simulink library "halin"  (R2021b)
settings: Solver=VariableStepAuto  StartTime=0.0  StopTime=10.0  RelTol=1e-3
undefined symbols (not defined in the file): KHAL_CAN1ABM1E2E_flg, KHAL_CAN1EPB1E2E_flg, KHAL_CAN1EPS1E2E_flg, KHAL_CAN1ESC1E2E_flg, KHAL_CAN1ESC5E2E_flg, KHAL_CAN3BMS1E2E_flg, KHAL_CAN3BMS6E2E_flg, KHAL_CAN3CCU1E2E_flg, KHAL_CAN3CCU2E2E_flg, KHAL_CAN3MCUNF1E2E_flg, KHAL_CAN3MCUNR1E2E_flg, KHAL_CAN3Shifter1E2E_flg, KHAL_CAN3Shifter2E2E_flg, KHAL_CAN6FCM2E2E_flg, KHAL_CAN6FCM4E2E_flg, TRUE
libraries: simulink x645, FVT_lib x212, hcu_lib x59
(part 14 of 23)

== system halin/HAL_IN/CAN3/VHAL_CANMsgInvalidMCUNF1_flg ==
  Cast To Boolean13 : DataTypeConversion  OutDataTypeStr=boolean
  Constant : Constant  Value=TRUE
  Latch13 : hcu_lib/Basic_Blocks/Latch
  Switch13 : Switch  Criteria=u2 ~= 0
  Unit Delay : UnitDelay  SampleTime=-1  HasFrameUpgradeWarning=on
  UnitConverter : DataTypeConversion  OutDataTypeStr=boolean
  Out : Outport
  wires:
  Constant/1 -> Switch13/3
  Unit Delay/1 -> Cast To Boolean13/1
  Cast To Boolean13/1 -> Switch13/1, Latch13/1
  Switch13/1 -> UnitConverter/1
  Latch13/1 -> Switch13/2
  UnitConverter/1 -> Unit Delay/1, Out/1  "VHAL_CANMsgInvalidMCUNF1_flg"

== system halin/HAL_IN/CAN3/VHAL_CANMsgInvalidMCUNF2_flg ==
  Cast To Boolean13 : DataTypeConversion  OutDataTypeStr=boolean
  Constant : Constant  Value=TRUE
  Latch13 : hcu_lib/Basic_Blocks/Latch
  Switch13 : Switch  Criteria=u2 ~= 0
  Unit Delay : UnitDelay  SampleTime=-1  HasFrameUpgradeWarning=on
  UnitConverter : DataTypeConversion  OutDataTypeStr=boolean
  Out : Outport
  wires:
  Constant/1 -> Switch13/3
  Unit Delay/1 -> Cast To Boolean13/1
  Cast To Boolean13/1 -> Switch13/1, Latch13/1
  Switch13/1 -> UnitConverter/1
  Latch13/1 -> Switch13/2
  UnitConverter/1 -> Unit Delay/1, Out/1  "VHAL_CANMsgInvalidMCUNF2_flg"

== system halin/HAL_IN/CAN3/VHAL_CANMsgInvalidMCUNF3_flg ==
  Cast To Boolean13 : DataTypeConversion  OutDataTypeStr=boolean
  Constant : Constant  Value=TRUE
  Latch13 : hcu_lib/Basic_Blocks/Latch
  Switch13 : Switch  Criteria=u2 ~= 0
  Unit Delay : UnitDelay  SampleTime=-1  HasFrameUpgradeWarning=on
  UnitConverter : DataTypeConversion  OutDataTypeStr=boolean
  Out : Outport
  wires:
  Constant/1 -> Switch13/3
  Unit Delay/1 -> Cast To Boolean13/1
  Cast To Boolean13/1 -> Switch13/1, Latch13/1
  Switch13/1 -> UnitConverter/1
  Latch13/1 -> Switch13/2
  UnitConverter/1 -> Unit Delay/1, Out/1  "VHAL_CANMsgInvalidMCUNF3_flg"

== system halin/HAL_IN/CAN3/VHAL_CANMsgInvalidMCUNR1_flg ==
  Cast To Boolean13 : DataTypeConversion  OutDataTypeStr=boolean
  Constant : Constant  Value=TRUE
  Latch13 : hcu_lib/Basic_Blocks/Latch
  Switch13 : Switch  Criteria=u2 ~= 0
  Unit Delay : UnitDelay  SampleTime=-1  HasFrameUpgradeWarning=on
  UnitConverter : DataTypeConversion  OutDataTypeStr=boolean
  Out : Outport
  wires:
  Constant/1 -> Switch13/3
  Unit Delay/1 -> Cast To Boolean13/1
  Cast To Boolean13/1 -> Switch13/1, Latch13/1
  Switch13/1 -> UnitConverter/1
  Latch13/1 -> Switch13/2
  UnitConverter/1 -> Unit Delay/1, Out/1  "VHAL_CANMsgInvalidMCUNR1_flg"

== system halin/HAL_IN/CAN3/VHAL_CANMsgInvalidMCUNR2_flg ==
  Cast To Boolean13 : DataTypeConversion  OutDataTypeStr=boolean
  Constant : Constant  Value=TRUE
  Latch13 : hcu_lib/Basic_Blocks/Latch
  Switch13 : Switch  Criteria=u2 ~= 0
  Unit Delay : UnitDelay  SampleTime=-1  HasFrameUpgradeWarning=on
  UnitConverter : DataTypeConversion  OutDataTypeStr=boolean
  Out : Outport
  wires:
  Constant/1 -> Switch13/3
  Unit Delay/1 -> Cast To Boolean13/1
  Cast To Boolean13/1 -> Switch13/1, Latch13/1
  Switch13/1 -> UnitConverter/1
  Latch13/1 -> Switch13/2
  UnitConverter/1 -> Unit Delay/1, Out/1  "VHAL_CANMsgInvalidMCUNR2_flg"

== system halin/HAL_IN/CAN3/VHAL_CANMsgInvalidMCUNR3_flg ==
  Cast To Boolean13 : DataTypeConversion  OutDataTypeStr=boolean
  Constant : Constant  Value=TRUE
  Latch13 : hcu_lib/Basic_Blocks/Latch
  Switch13 : Switch  Criteria=u2 ~= 0
  Unit Delay : UnitDelay  SampleTime=-1  HasFrameUpgradeWarning=on
  UnitConverter : DataTypeConversion  OutDataTypeStr=boolean
  Out : Outport
  wires:
  Constant/1 -> Switch13/3
  Unit Delay/1 -> Cast To Boolean13/1
  Cast To Boolean13/1 -> Switch13/1, Latch13/1
  Switch13/1 -> UnitConverter/1
  Latch13/1 -> Switch13/2
  UnitConverter/1 -> Unit Delay/1, Out/1  "VHAL_CANMsgInvalidMCUNR3_flg"

== system halin/HAL_IN/CAN3/VHAL_CANMsgInvalidShifter1_flg ==
  Cast To Boolean13 : DataTypeConversion  OutDataTypeStr=boolean
  Constant : Constant  Value=TRUE
  Latch13 : hcu_lib/Basic_Blocks/Latch
  Switch13 : Switch  Criteria=u2 ~= 0
  Unit Delay : UnitDelay  SampleTime=-1  HasFrameUpgradeWarning=on
  UnitConverter : DataTypeConversion  OutDataTypeStr=boolean
  Out : Outport
  wires:
  Constant/1 -> Switch13/3
  Unit Delay/1 -> Cast To Boolean13/1
  Cast To Boolean13/1 -> Switch13/1, Latch13/1
  Switch13/1 -> UnitConverter/1
  Latch13/1 -> Switch13/2
  UnitConverter/1 -> Unit Delay/1, Out/1  "VHAL_CANMsgInvalidShifter1_flg"

== system halin/HAL_IN/CAN3/VHAL_CANMsgInvalidShifter2_flg ==
  Cast To Boolean13 : DataTypeConversion  OutDataTypeStr=boolean
  Constant : Constant  Value=TRUE
  Latch13 : hcu_lib/Basic_Blocks/Latch
  Switch13 : Switch  Criteria=u2 ~= 0
  Unit Delay : UnitDelay  SampleTime=-1  HasFrameUpgradeWarning=on
  UnitConverter : DataTypeConversion  OutDataTypeStr=boolean
  Out : Outport
  wires:
  Constant/1 -> Switch13/3
  Unit Delay/1 -> Cast To Boolean13/1
  Cast To Boolean13/1 -> Switch13/1, Latch13/1
  Switch13/1 -> UnitConverter/1
  Latch13/1 -> Switch13/2
  UnitConverter/1 -> Unit Delay/1, Out/1  "VHAL_CANMsgInvalidShifter2_flg"

== system halin/HAL_IN/CAN4/BodyZone_DR1 ==
  DT_CAN4_SG_BodyZone_DR1 : Inport
  BDDSEATAntiSta : Subsystem
  BDDSEATEntryFunSta : Subsystem
  BDDSEATErrorSta : Subsystem
  BDDSEATMemSetSta : Subsystem
  BDDSEATModeSta : Subsystem
  BDDSEATVentSta : Subsystem
  BDDSEATheaterSta : Subsystem
  bus_selector : BusSelector  OutputSignals=CAN4_BD_DSEAT_Anti_Sta
  bus_selector1 : BusSelector  OutputSignals=CAN4_BD_DSEAT_EntryFun_Sta
  bus_selector2 : BusSelector  OutputSignals=CAN4_BD_DSEAT_Error_Sta
  bus_selector3 : BusSelector  OutputSignals=CAN4_BD_DSEAT_MemSet_Sta
  bus_selector4 : BusSelector  OutputSignals=CAN4_BD_DSEAT_Mode_Sta
  bus_selector5 : BusSelector  OutputSignals=CAN4_BD_DSEAT_Vent_Sta
  bus_selector6 : BusSelector  OutputSignals=CAN4_BD_DSEAT_heater_Sta
  VHAL_BDDSEATAntiSta_flg : Outport
  VHAL_BDDSEATEntryFunSta_flg : Outport  Port=2
  VHAL_BDDSEATErrorSta_flg : Outport  Port=3
  VHAL_BDDSEATMemSetSta_enum : Outport  Port=4
  VHAL_BDDSEATModeSta_enum : Outport  Port=5
  VHAL_BDDSEATVentSta_enum : Outport  Port=6
  VHAL_BDDSEATheaterSta_enum : Outport  Port=7
  wires:
  DT_CAN4_SG_BodyZone_DR1/1 -> [DT_CAN4_SG_BodyZone_DR1]
  [DT_CAN4_SG_BodyZone_DR1] -> bus_selector/1
  bus_selector/1 -> BDDSEATAntiSta/1(BD_DSEAT_Anti_Sta)  "<CAN4_BD_DSEAT_Anti_Sta>"
  BDDSEATAntiSta/1(VHAL_BDDSEATAntiSta_flg) -> VHAL_BDDSEATAntiSta_flg/1
  [DT_CAN4_SG_BodyZone_DR1] -> bus_selector1/1
  bus_selector1/1 -> BDDSEATEntryFunSta/1(BD_DSEAT_EntryFun_Sta)  "<CAN4_BD_DSEAT_EntryFun_Sta>"
  BDDSEATEntryFunSta/1(VHAL_BDDSEATEntryFunSta_flg) -> VHAL_BDDSEATEntryFunSta_flg/1
  [DT_CAN4_SG_BodyZone_DR1] -> bus_selector2/1
  bus_selector2/1 -> BDDSEATErrorSta/1(BD_DSEAT_Error_Sta)  "<CAN4_BD_DSEAT_Error_Sta>"
  BDDSEATErrorSta/1(VHAL_BDDSEATErrorSta_flg) -> VHAL_BDDSEATErrorSta_flg/1
  [DT_CAN4_SG_BodyZone_DR1] -> bus_selector3/1
  bus_selector3/1 -> BDDSEATMemSetSta/1(BD_DSEAT_MemSet_Sta)  "<CAN4_BD_DSEAT_MemSet_Sta>"
  BDDSEATMemSetSta/1(VHAL_BDDSEATMemSetSta_enum) -> VHAL_BDDSEATMemSetSta_enum/1
  [DT_CAN4_SG_BodyZone_DR1] -> bus_selector4/1
  bus_selector4/1 -> BDDSEATModeSta/1(BD_DSEAT_Mode_Sta)  "<CAN4_BD_DSEAT_Mode_Sta>"
  BDDSEATModeSta/1(VHAL_BDDSEATModeSta_enum) -> VHAL_BDDSEATModeSta_enum/1
  [DT_CAN4_SG_BodyZone_DR1] -> bus_selector5/1
  bus_selector5/1 -> BDDSEATVentSta/1(BD_DSEAT_Vent_Sta)  "<CAN4_BD_DSEAT_Vent_Sta>"
  BDDSEATVentSta/1(VHAL_BDDSEATVentSta_enum) -> VHAL_BDDSEATVentSta_enum/1
  [DT_CAN4_SG_BodyZone_DR1] -> bus_selector6/1
  bus_selector6/1 -> BDDSEATheaterSta/1(BD_DSEAT_heater_Sta)  "<CAN4_BD_DSEAT_heater_Sta>"
  BDDSEATheaterSta/1(VHAL_BDDSEATheaterSta_enum) -> VHAL_BDDSEATheaterSta_enum/1

== system halin/HAL_IN/CAN4/BodyZone_DR2 ==
  DT_CAN4_SG_BodyZone_DR2 : Inport
  BDAPMWinFOpenedSta : Subsystem
  BDAPMWinROpenedSta : Subsystem
  BDDoorFHandleCloseSta : Subsystem
  BDDoorRHandleCloseSta : Subsystem
  bus_selector : BusSelector  OutputSignals=CAN4_BD_APM_WinFOpened_Sta
  bus_selector1 : BusSelector  OutputSignals=CAN4_BD_APM_WinROpened_Sta
  bus_selector2 : BusSelector  OutputSignals=CAN4_BD_Door_FHandleClose_Sta
  bus_selector3 : BusSelector  OutputSignals=CAN4_BD_Door_RHandleClose_Sta
  VHAL_BDAPMWinFOpenedSta_pct : Outport
  VHAL_BDAPMWinROpenedSta_pct : Outport  Port=2
  VHAL_BDDoorFHandleCloseSta_flg : Outport  Port=3
  VHAL_BDDoorRHandleCloseSta_flg : Outport  Port=4
  wires:
  DT_CAN4_SG_BodyZone_DR2/1 -> [DT_CAN4_SG_BodyZone_DR2]
  [DT_CAN4_SG_BodyZone_DR2] -> bus_selector/1
  bus_selector/1 -> BDAPMWinFOpenedSta/1(BD_APM_WinFOpened_Sta)  "<CAN4_BD_APM_WinFOpened_Sta>"
  BDAPMWinFOpenedSta/1(VHAL_BDAPMWinFOpenedSta_pct) -> VHAL_BDAPMWinFOpenedSta_pct/1
  [DT_CAN4_SG_BodyZone_DR2] -> bus_selector1/1
  bus_selector1/1 -> BDAPMWinROpenedSta/1(BD_APM_WinROpened_Sta)  "<CAN4_BD_APM_WinROpened_Sta>"
  BDAPMWinROpenedSta/1(VHAL_BDAPMWinROpenedSta_pct) -> VHAL_BDAPMWinROpenedSta_pct/1
  [DT_CAN4_SG_BodyZone_DR2] -> bus_selector2/1
  bus_selector2/1 -> BDDoorFHandleCloseSta/1(BD_Door_FHandleClose_Sta)  "<CAN4_BD_Door_FHandleClose_Sta>"
  BDDoorFHandleCloseSta/1(VHAL_BDDoorFHandleCloseSta_flg) -> VHAL_BDDoorFHandleCloseSta_flg/1
  [DT_CAN4_SG_BodyZone_DR2] -> bus_selector3/1
  bus_selector3/1 -> BDDoorRHandleCloseSta/1(BD_Door_RHandleClose_Sta)  "<CAN4_BD_Door_RHandleClose_Sta>"
  BDDoorRHandleCloseSta/1(VHAL_BDDoorRHandleCloseSta_flg) -> VHAL_BDDoorRHandleCloseSta_flg/1

== system halin/HAL_IN/CAN4/BodyZone_PS1 ==
  DT_CAN4_SG_BodyZone_PS1 : Inport
  BPPSEATErrorSta : Subsystem
  BPPSEATModeSta : Subsystem
  BPPSEATVentSta : Subsystem
  BPPSEATheaterSta : Subsystem
  BPPTGActiveSta : Subsystem
  BPPTGExistSta : Subsystem
  BPPTGInsideSW1Sta : Subsystem
  BPPTGInsideSW2Sta : Subsystem
  BPPTGIsSetHeightSta : Subsystem
  BPPTGLeftHallPosnSta : Subsystem
  BPPTGOpenRatioSta : Subsystem
  BPPTGRDILCmd : Subsystem
  BPPTGSysSta : Subsystem
  bus_selector : BusSelector  OutputSignals=CAN4_BP_PSEAT_Error_Sta
  bus_selector1 : BusSelector  OutputSignals=CAN4_BP_PSEAT_Mode_Sta
  bus_selector10 : BusSelector  OutputSignals=CAN4_BP_PTG_OpenRatio_Sta
  bus_selector11 : BusSelector  OutputSignals=CAN4_BP_PTG_RDIL_Cmd
  bus_selector12 : BusSelector  OutputSignals=CAN4_BP_PTG_Sys_Sta
  bus_selector2 : BusSelector  OutputSignals=CAN4_BP_PSEAT_Vent_Sta
  bus_selector3 : BusSelector  OutputSignals=CAN4_BP_PSEAT_heater_Sta
  bus_selector4 : BusSelector  OutputSignals=CAN4_BP_PTG_Active_Sta
  bus_selector5 : BusSelector  OutputSignals=CAN4_BP_PTG_Exist_Sta
  bus_selector6 : BusSelector  OutputSignals=CAN4_BP_PTG_InsideSW1_Sta
  bus_selector7 : BusSelector  OutputSignals=CAN4_BP_PTG_InsideSW2_Sta
  bus_selector8 : BusSelector  OutputSignals=CAN4_BP_PTG_IsSetHeight_Sta
  bus_selector9 : BusSelector  OutputSignals=CAN4_BP_PTG_LeftHallPosn_Sta
  VHAL_BPPSEATErrorSta_flg : Outport
  VHAL_BPPSEATModeSta_enum : Outport  Port=2
  VHAL_BPPSEATVentSta_enum : Outport  Port=3
  VHAL_BPPSEATheaterSta_enum : Outport  Port=4
  VHAL_BPPTGActiveSta_enum : Outport  Port=5
  VHAL_BPPTGExistSta_flg : Outport  Port=6
  VHAL_BPPTGInsideSW1Sta_enum : Outport  Port=7
  VHAL_BPPTGInsideSW2Sta_enum : Outport  Port=8
  VHAL_BPPTGIsSetHeightSta_flg : Outport  Port=9
  VHAL_BPPTGLeftHallPosnSta_enum : Outport  Port=10
  VHAL_BPPTGOpenRatioSta_pct : Outport  Port=11
  VHAL_BPPTGRDILCmd_enum : Outport  Port=12
  VHAL_BPPTGSysSta_enum : Outport  Port=13
  wires:
  DT_CAN4_SG_BodyZone_PS1/1 -> [DT_CAN4_SG_BodyZone_PS1]
  [DT_CAN4_SG_BodyZone_PS1] -> bus_selector/1
  bus_selector/1 -> BPPSEATErrorSta/1(BP_PSEAT_Error_Sta)  "<CAN4_BP_PSEAT_Error_Sta>"
  BPPSEATErrorSta/1(VHAL_BPPSEATErrorSta_flg) -> VHAL_BPPSEATErrorSta_flg/1
  [DT_CAN4_SG_BodyZone_PS1] -> bus_selector1/1
  bus_selector1/1 -> BPPSEATModeSta/1(BP_PSEAT_Mode_Sta)  "<CAN4_BP_PSEAT_Mode_Sta>"
  BPPSEATModeSta/1(VHAL_BPPSEATModeSta_enum) -> VHAL_BPPSEATModeSta_enum/1
  [DT_CAN4_SG_BodyZone_PS1] -> bus_selector2/1
  bus_selector2/1 -> BPPSEATVentSta/1(BP_PSEAT_Vent_Sta)  "<CAN4_BP_PSEAT_Vent_Sta>"
  BPPSEATVentSta/1(VHAL_BPPSEATVentSta_enum) -> VHAL_BPPSEATVentSta_enum/1
  [DT_CAN4_SG_BodyZone_PS1] -> bus_selector3/1
  bus_selector3/1 -> BPPSEATheaterSta/1(BP_PSEAT_heater_Sta)  "<CAN4_BP_PSEAT_heater_Sta>"
  BPPSEATheaterSta/1(VHAL_BPPSEATheaterSta_enum) -> VHAL_BPPSEATheaterSta_enum/1
  [DT_CAN4_SG_BodyZone_PS1] -> bus_selector4/1
  bus_selector4/1 -> BPPTGActiveSta/1(BP_PTG_Active_Sta)  "<CAN4_BP_PTG_Active_Sta>"
  BPPTGActiveSta/1(VHAL_BPPTGActiveSta_enum) -> VHAL_BPPTGActiveSta_enum/1
  [DT_CAN4_SG_BodyZone_PS1] -> bus_selector5/1
  bus_selector5/1 -> BPPTGExistSta/1(BP_PTG_Exist_Sta)  "<CAN4_BP_PTG_Exist_Sta>"
  BPPTGExistSta/1(VHAL_BPPTGExistSta_flg) -> VHAL_BPPTGExistSta_flg/1
  [DT_CAN4_SG_BodyZone_PS1] -> bus_selector6/1
  bus_selector6/1 -> BPPTGInsideSW1Sta/1(BP_PTG_InsideSW1_Sta)  "<CAN4_BP_PTG_InsideSW1_Sta>"
  BPPTGInsideSW1Sta/1(VHAL_BPPTGInsideSW1Sta_enum) -> VHAL_BPPTGInsideSW1Sta_enum/1
  [DT_CAN4_SG_BodyZone_PS1] -> bus_selector7/1
  bus_selector7/1 -> BPPTGInsideSW2Sta/1(BP_PTG_InsideSW2_Sta)  "<CAN4_BP_PTG_InsideSW2_Sta>"
  BPPTGInsideSW2Sta/1(VHAL_BPPTGInsideSW2Sta_enum) -> VHAL_BPPTGInsideSW2Sta_enum/1
  [DT_CAN4_SG_BodyZone_PS1] -> bus_selector8/1
  bus_selector8/1 -> BPPTGIsSetHeightSta/1(BP_PTG_IsSetHeight_Sta)  "<CAN4_BP_PTG_IsSetHeight_Sta>"
  BPPTGIsSetHeightSta/1(VHAL_BPPTGIsSetHeightSta_flg) -> VHAL_BPPTGIsSetHeightSta_flg/1
  [DT_CAN4_SG_BodyZone_PS1] -> bus_selector9/1
  bus_selector9/1 -> BPPTGLeftHallPosnSta/1(BP_PTG_LeftHallPosn_Sta)  "<CAN4_BP_PTG_LeftHallPosn_Sta>"
  BPPTGLeftHallPosnSta/1(VHAL_BPPTGLeftHallPosnSta_enum) -> VHAL_BPPTGLeftHallPosnSta_enum/1
  [DT_CAN4_SG_BodyZone_PS1] -> bus_selector10/1
  bus_selector10/1 -> BPPTGOpenRatioSta/1(BP_PTG_OpenRatio_Sta)  "<CAN4_BP_PTG_OpenRatio_Sta>"
  BPPTGOpenRatioSta/1(VHAL_BPPTGOpenRatioSta_pct) -> VHAL_BPPTGOpenRatioSta_pct/1
  [DT_CAN4_SG_BodyZone_PS1] -> bus_selector11/1
  bus_selector11/1 -> BPPTGRDILCmd/1(BP_PTG_RDIL_Cmd)  "<CAN4_BP_PTG_RDIL_Cmd>"
  BPPTGRDILCmd/1(VHAL_BPPTGRDILCmd_enum) -> VHAL_BPPTGRDILCmd_enum/1
  [DT_CAN4_SG_BodyZone_PS1] -> bus_selector12/1
  bus_selector12/1 -> BPPTGSysSta/1(BP_PTG_Sys_Sta)  "<CAN4_BP_PTG_Sys_Sta>"
  BPPTGSysSta/1(VHAL_BPPTGSysSta_enum) -> VHAL_BPPTGSysSta_enum/1

== system halin/HAL_IN/CAN4/BodyZone_PS2 ==
  DT_CAN4_SG_BodyZone_PS2 : Inport
  BPAPMWinFOpenedSta : Subsystem
  BPAPMWinROpenedSta : Subsystem
  BPDoorFHandleCloseSta : Subsystem
  BPDoorRHandleCloseSta : Subsystem
  BPSEATLVentSta : Subsystem
  BPSEATMLVentSta : Subsystem
  BPSEATMRVentSta : Subsystem
  BPSEATRVentSta : Subsystem
  bus_selector : BusSelector  OutputSignals=CAN4_BP_APM_WinFOpened_Sta
  bus_selector1 : BusSelector  OutputSignals=CAN4_BP_APM_WinROpened_Sta
  bus_selector2 : BusSelector  OutputSignals=CAN4_BP_Door_FHandleClose_Sta
  bus_selector3 : BusSelector  OutputSignals=CAN4_BP_Door_RHandleClose_Sta
  bus_selector4 : BusSelector  OutputSignals=CAN4_BP_SEAT_LVent_Sta
  bus_selector5 : BusSelector  OutputSignals=CAN4_BP_SEAT_MLVent_Sta
  bus_selector6 : BusSelector  OutputSignals=CAN4_BP_SEAT_MRVent_Sta
  bus_selector7 : BusSelector  OutputSignals=CAN4_BP_SEAT_RVent_Sta
  VHAL_BPAPMWinFOpenedSta_pct : Outport
  VHAL_BPAPMWinROpenedSta_pct : Outport  Port=2
  VHAL_BPDoorFHandleCloseSta_flg : Outport  Port=3
  VHAL_BPDoorRHandleCloseSta_flg : Outport  Port=4
  VHAL_BPSEATLVentSta_enum : Outport  Port=5
  VHAL_BPSEATMLVentSta_enum : Outport  Port=6
  VHAL_BPSEATMRVentSta_enum : Outport  Port=7
  VHAL_BPSEATRVentSta_enum : Outport  Port=8
  wires:
  DT_CAN4_SG_BodyZone_PS2/1 -> [DT_CAN4_SG_BodyZone_PS2]
  [DT_CAN4_SG_BodyZone_PS2] -> bus_selector/1
  bus_selector/1 -> BPAPMWinFOpenedSta/1(BP_APM_WinFOpened_Sta)  "<CAN4_BP_APM_WinFOpened_Sta>"
  BPAPMWinFOpenedSta/1(VHAL_BPAPMWinFOpenedSta_pct) -> VHAL_BPAPMWinFOpenedSta_pct/1
  [DT_CAN4_SG_BodyZone_PS2] -> bus_selector1/1
  bus_selector1/1 -> BPAPMWinROpenedSta/1(BP_APM_WinROpened_Sta)  "<CAN4_BP_APM_WinROpened_Sta>"
  BPAPMWinROpenedSta/1(VHAL_BPAPMWinROpenedSta_pct) -> VHAL_BPAPMWinROpenedSta_pct/1
  [DT_CAN4_SG_BodyZone_PS2] -> bus_selector2/1
  bus_selector2/1 -> BPDoorFHandleCloseSta/1(BP_Door_FHandleClose_Sta)  "<CAN4_BP_Door_FHandleClose_Sta>"
  BPDoorFHandleCloseSta/1(VHAL_BPDoorFHandleCloseSta_flg) -> VHAL_BPDoorFHandleCloseSta_flg/1
  [DT_CAN4_SG_BodyZone_PS2] -> bus_selector3/1
  bus_selector3/1 -> BPDoorRHandleCloseSta/1(BP_Door_RHandleClose_Sta)  "<CAN4_BP_Door_RHandleClose_Sta>"
  BPDoorRHandleCloseSta/1(VHAL_BPDoorRHandleCloseSta_flg) -> VHAL_BPDoorRHandleCloseSta_flg/1
  [DT_CAN4_SG_BodyZone_PS2] -> bus_selector4/1
  bus_selector4/1 -> BPSEATLVentSta/1(BP_SEAT_LVent_Sta)  "<CAN4_BP_SEAT_LVent_Sta>"
  BPSEATLVentSta/1(VHAL_BPSEATLVentSta_enum) -> VHAL_BPSEATLVentSta_enum/1
  [DT_CAN4_SG_BodyZone_PS2] -> bus_selector5/1
  bus_selector5/1 -> BPSEATMLVentSta/1(BP_SEAT_MLVent_Sta)  "<CAN4_BP_SEAT_MLVent_Sta>"
  BPSEATMLVentSta/1(VHAL_BPSEATMLVentSta_enum) -> VHAL_BPSEATMLVentSta_enum/1
  [DT_CAN4_SG_BodyZone_PS2] -> bus_selector6/1
  bus_selector6/1 -> BPSEATMRVentSta/1(BP_SEAT_MRVent_Sta)  "<CAN4_BP_SEAT_MRVent_Sta>"
  BPSEATMRVentSta/1(VHAL_BPSEATMRVentSta_enum) -> VHAL_BPSEATMRVentSta_enum/1
  [DT_CAN4_SG_BodyZone_PS2] -> bus_selector7/1
  bus_selector7/1 -> BPSEATRVentSta/1(BP_SEAT_RVent_Sta)  "<CAN4_BP_SEAT_RVent_Sta>"
  BPSEATRVentSta/1(VHAL_BPSEATRVentSta_enum) -> VHAL_BPSEATRVentSta_enum/1

== system halin/HAL_IN/CAN4/DKC1 ==
  DT_CAN4_SG_DKC1 : Inport
  DKCKeyNumSta : Subsystem
  DKCKeyTypeSta : Subsystem
  DKCPDkeyAreaRAPSSta : Subsystem
  DKCParkingModeCmd : Subsystem
  DKCReVehData : Subsystem
  PCommandToBCM : Subsystem
  PCommandToPTG : Subsystem
  PDKeyAreaLockUnlock : Subsystem
  PDKeyAreaPS : Subsystem
  PDKeyAreaPTG : Subsystem
  PDKeyWelcome : Subsystem
  PDkeyShowIVI : Subsystem
  PKeyMiss : Subsystem
  PKeyMode : Subsystem
  PUIDLowPower : Subsystem
  bus_selector : BusSelector  OutputSignals=CAN4_DKC_KeyNum_Sta
  bus_selector1 : BusSelector  OutputSignals=CAN4_DKC_KeyType_Sta
  bus_selector10 : BusSelector  OutputSignals=CAN4_P_DKey_Welcome
  bus_selector11 : BusSelector  OutputSignals=CAN4_P_Dkey_Show_IVI
  bus_selector12 : BusSelector  OutputSignals=CAN4_P_KeyMiss
  bus_selector13 : BusSelector  OutputSignals=CAN4_P_KeyMode
  bus_selector14 : BusSelector  OutputSignals=CAN4_P_UID_LowPower
  bus_selector2 : BusSelector  OutputSignals=CAN4_DKC_PDkeyAreaRAPS_Sta
  bus_selector3 : BusSelector  OutputSignals=CAN4_DKC_ParkingMode_Cmd
  bus_selector4 : BusSelector  OutputSignals=CAN4_DKC_Re_VehData
  bus_selector5 : BusSelector  OutputSignals=CAN4_P_CommandToBCM
  bus_selector6 : BusSelector  OutputSignals=CAN4_P_CommandToPTG
  bus_selector7 : BusSelector  OutputSignals=CAN4_P_DKey_Area_LockUnlock
  bus_selector8 : BusSelector  OutputSignals=CAN4_P_DKey_Area_PS
  bus_selector9 : BusSelector  OutputSignals=CAN4_P_DKey_Area_PTG
  VHAL_DKCKeyNumSta_enum : Outport
  VHAL_DKCKeyTypeSta_enum : Outport  Port=2
  VHAL_DKCPDkeyAreaRAPSSta_enum : Outport  Port=3
  VHAL_DKCParkingModeCmd_enum : Outport  Port=4
  VHAL_DKCReVehData_enum : Outport  Port=5
  VHAL_PCommandToBCM_enum : Outport  Port=6
  VHAL_PCommandToPTG_enum : Outport  Port=7
  VHAL_PDKeyAreaLockUnlock_enum : Outport  Port=8
  VHAL_PDKeyAreaPS_enum : Outport  Port=9
  VHAL_PDKeyAreaPTG_enum : Outport  Port=10
  VHAL_PDKeyWelcome_enum : Outport  Port=11
  VHAL_PDkeyShowIVI_enum : Outport  Port=12
  VHAL_PKeyMiss_flg : Outport  Port=13
  VHAL_PKeyMode_enum : Outport  Port=14
  VHAL_PUIDLowPower_flg : Outport  Port=15
  wires:
  DT_CAN4_SG_DKC1/1 -> [DT_CAN4_SG_DKC1]
  [DT_CAN4_SG_DKC1] -> bus_selector/1
  bus_selector/1 -> DKCKeyNumSta/1(DKC_KeyNum_Sta)  "<CAN4_DKC_KeyNum_Sta>"
  DKCKeyNumSta/1(VHAL_DKCKeyNumSta_enum) -> VHAL_DKCKeyNumSta_enum/1
  [DT_CAN4_SG_DKC1] -> bus_selector1/1
  bus_selector1/1 -> DKCKeyTypeSta/1(DKC_KeyType_Sta)  "<CAN4_DKC_KeyType_Sta>"
  DKCKeyTypeSta/1(VHAL_DKCKeyTypeSta_enum) -> VHAL_DKCKeyTypeSta_enum/1
  [DT_CAN4_SG_DKC1] -> bus_selector2/1
  bus_selector2/1 -> DKCPDkeyAreaRAPSSta/1(DKC_PDkeyAreaRAPS_Sta)  "<CAN4_DKC_PDkeyAreaRAPS_Sta>"
  DKCPDkeyAreaRAPSSta/1(VHAL_DKCPDkeyAreaRAPSSta_enum) -> VHAL_DKCPDkeyAreaRAPSSta_enum/1
  [DT_CAN4_SG_DKC1] -> bus_selector3/1
  bus_selector3/1 -> DKCParkingModeCmd/1(DKC_ParkingMode_Cmd)  "<CAN4_DKC_ParkingMode_Cmd>"
  DKCParkingModeCmd/1(VHAL_DKCParkingModeCmd_enum) -> VHAL_DKCParkingModeCmd_enum/1
  [DT_CAN4_SG_DKC1] -> bus_selector4/1
  bus_selector4/1 -> DKCReVehData/1(DKC_Re_VehData)  "<CAN4_DKC_Re_VehData>"
  DKCReVehData/1(VHAL_DKCReVehData_enum) -> VHAL_DKCReVehData_enum/1
  [DT_CAN4_SG_DKC1] -> bus_selector5/1
  bus_selector5/1 -> PCommandToBCM/1(P_CommandToBCM)  "<CAN4_P_CommandToBCM>"
  PCommandToBCM/1(VHAL_PCommandToBCM_enum) -> VHAL_PCommandToBCM_enum/1
  [DT_CAN4_SG_DKC1] -> bus_selector6/1
  bus_selector6/1 -> PCommandToPTG/1(P_CommandToPTG)  "<CAN4_P_CommandToPTG>"
  PCommandToPTG/1(VHAL_PCommandToPTG_enum) -> VHAL_PCommandToPTG_enum/1
  [DT_CAN4_SG_DKC1] -> bus_selector7/1
  bus_selector7/1 -> PDKeyAreaLockUnlock/1(P_DKey_Area_LockUnlock)  "<CAN4_P_DKey_Area_LockUnlock>"
  PDKeyAreaLockUnlock/1(VHAL_PDKeyAreaLockUnlock_enum) -> VHAL_PDKeyAreaLockUnlock_enum/1
  [DT_CAN4_SG_DKC1] -> bus_selector8/1
  bus_selector8/1 -> PDKeyAreaPS/1(P_DKey_Area_PS)  "<CAN4_P_DKey_Area_PS>"
  PDKeyAreaPS/1(VHAL_PDKeyAreaPS_enum) -> VHAL_PDKeyAreaPS_enum/1
  [DT_CAN4_SG_DKC1] -> bus_selector9/1
  bus_selector9/1 -> PDKeyAreaPTG/1(P_DKey_Area_PTG)  "<CAN4_P_DKey_Area_PTG>"
  PDKeyAreaPTG/1(VHAL_PDKeyAreaPTG_enum) -> VHAL_PDKeyAreaPTG_enum/1
  [DT_CAN4_SG_DKC1] -> bus_selector10/1
  bus_selector10/1 -> PDKeyWelcome/1(P_DKey_Welcome)  "<CAN4_P_DKey_Welcome>"
  PDKeyWelcome/1(VHAL_PDKeyWelcome_enum) -> VHAL_PDKeyWelcome_enum/1
  [DT_CAN4_SG_DKC1] -> bus_selector11/1
  bus_selector11/1 -> PDkeyShowIVI/1(P_Dkey_Show_IVI)  "<CAN4_P_Dkey_Show_IVI>"
  PDkeyShowIVI/1(VHAL_PDkeyShowIVI_enum) -> VHAL_PDkeyShowIVI_enum/1
  [DT_CAN4_SG_DKC1] -> bus_selector12/1
  bus_selector12/1 -> PKeyMiss/1(P_KeyMiss)  "<CAN4_P_KeyMiss>"
  PKeyMiss/1(VHAL_PKeyMiss_flg) -> VHAL_PKeyMiss_flg/1
  [DT_CAN4_SG_DKC1] -> bus_selector13/1
  bus_selector13/1 -> PKeyMode/1(P_KeyMode)  "<CAN4_P_KeyMode>"
  PKeyMode/1(VHAL_PKeyMode_enum) -> VHAL_PKeyMode_enum/1
  [DT_CAN4_SG_DKC1] -> bus_selector14/1
  bus_selector14/1 -> PUIDLowPower/1(P_UID_LowPower)  "<CAN4_P_UID_LowPower>"
  PUIDLowPower/1(VHAL_PUIDLowPower_flg) -> VHAL_PUIDLowPower_flg/1

== system halin/HAL_IN/CAN4/DKC2 ==
  DT_CAN4_SG_DKC2 : Inport
  EncryptionDATA063 : Subsystem
  EncryptionDATA64127 : Subsystem
  RandomNumberX : Subsystem
  bus_selector : BusSelector  OutputSignals=CAN4_EncryptionDATA_0_63
  bus_selector1 : BusSelector  OutputSignals=CAN4_EncryptionDATA_64_127
  bus_selector2 : BusSelector  OutputSignals=CAN4_Random_Number_X
  VHAL_EncryptionDATA063_enum : Outport
  VHAL_EncryptionDATA64127_enum : Outport  Port=2
  VHAL_RandomNumberX_enum : Outport  Port=3
  wires:
  DT_CAN4_SG_DKC2/1 -> [DT_CAN4_SG_DKC2]
  [DT_CAN4_SG_DKC2] -> bus_selector/1
  bus_selector/1 -> EncryptionDATA063/1(EncryptionDATA_0_63)  "<CAN4_EncryptionDATA_0_63>"
  EncryptionDATA063/1(VHAL_EncryptionDATA063_enum) -> VHAL_EncryptionDATA063_enum/1
  [DT_CAN4_SG_DKC2] -> bus_selector1/1
  bus_selector1/1 -> EncryptionDATA64127/1(EncryptionDATA_64_127)  "<CAN4_EncryptionDATA_64_127>"
  EncryptionDATA64127/1(VHAL_EncryptionDATA64127_enum) -> VHAL_EncryptionDATA64127_enum/1
  [DT_CAN4_SG_DKC2] -> bus_selector2/1
  bus_selector2/1 -> RandomNumberX/1(Random_Number_X)  "<CAN4_Random_Number_X>"
  RandomNumberX/1(VHAL_RandomNumberX_enum) -> VHAL_RandomNumberX_enum/1

== system halin/HAL_IN/CAN4/PTG1 ==
  DT_CAN4_SG_PTG1 : Inport
  PTGActiveSta : Subsystem
  PTGAutoStaus : Subsystem
  PTGExist : Subsystem
  PTGHWVer : Subsystem
  PTGInnerSW2 : Subsystem
  PTGIsSetHeight : Subsystem
  PTGOpenRatio : Subsystem
  PTGRDILSta : Subsystem
  PTGSWVer : Subsystem
  PTGSysSta : Subsystem
  bus_selector : BusSelector  OutputSignals=CAN4_PTG_Active_Sta
  bus_selector1 : BusSelector  OutputSignals=CAN4_PTG_AutoStaus
  bus_selector2 : BusSelector  OutputSignals=CAN4_PTG_Exist
  bus_selector3 : BusSelector  OutputSignals=CAN4_PTG_HW_Ver
  bus_selector4 : BusSelector  OutputSignals=CAN4_PTG_Inner_SW_2
  bus_selector5 : BusSelector  OutputSignals=CAN4_PTG_Is_Set_Height
  bus_selector6 : BusSelector  OutputSignals=CAN4_PTG_Open_Ratio
  bus_selector7 : BusSelector  OutputSignals=CAN4_PTG_RDIL_Sta
  bus_selector8 : BusSelector  OutputSignals=CAN4_PTG_SW_Ver
  bus_selector9 : BusSelector  OutputSignals=CAN4_PTG_Sys_Sta
  VHAL_PTGActiveSta_enum : Outport
  VHAL_PTGAutoStaus_flg : Outport  Port=2
  VHAL_PTGExist_flg : Outport  Port=3
  VHAL_PTGHWVer_enum : Outport  Port=4
  VHAL_PTGInnerSW2_enum : Outport  Port=5
  VHAL_PTGIsSetHeight_flg : Outport  Port=6
  VHAL_PTGOpenRatio_pct : Outport  Port=7
  VHAL_PTGRDILSta_enum : Outport  Port=8
  VHAL_PTGSWVer_enum : Outport  Port=9
  VHAL_PTGSysSta_enum : Outport  Port=10
  wires:
  DT_CAN4_SG_PTG1/1 -> [DT_CAN4_SG_PTG1]
  [DT_CAN4_SG_PTG1] -> bus_selector/1
  bus_selector/1 -> PTGActiveSta/1(PTG_Active_Sta)  "<CAN4_PTG_Active_Sta>"
  PTGActiveSta/1(VHAL_PTGActiveSta_enum) -> VHAL_PTGActiveSta_enum/1
  [DT_CAN4_SG_PTG1] -> bus_selector1/1
  bus_selector1/1 -> PTGAutoStaus/1(PTG_AutoStaus)  "<CAN4_PTG_AutoStaus>"
  PTGAutoStaus/1(VHAL_PTGAutoStaus_flg) -> VHAL_PTGAutoStaus_flg/1
  [DT_CAN4_SG_PTG1] -> bus_selector2/1
  bus_selector2/1 -> PTGExist/1(PTG_Exist)  "<CAN4_PTG_Exist>"
  PTGExist/1(VHAL_PTGExist_flg) -> VHAL_PTGExist_flg/1
  [DT_CAN4_SG_PTG1] -> bus_selector3/1
  bus_selector3/1 -> PTGHWVer/1(PTG_HW_Ver)  "<CAN4_PTG_HW_Ver>"
  PTGHWVer/1(VHAL_PTGHWVer_enum) -> VHAL_PTGHWVer_enum/1
  [DT_CAN4_SG_PTG1] -> bus_selector4/1
  bus_selector4/1 -> PTGInnerSW2/1(PTG_Inner_SW_2)  "<CAN4_PTG_Inner_SW_2>"
  PTGInnerSW2/1(VHAL_PTGInnerSW2_enum) -> VHAL_PTGInnerSW2_enum/1
  [DT_CAN4_SG_PTG1] -> bus_selector5/1
  bus_selector5/1 -> PTGIsSetHeight/1(PTG_Is_Set_Height)  "<CAN4_PTG_Is_Set_Height>"
  PTGIsSetHeight/1(VHAL_PTGIsSetHeight_flg) -> VHAL_PTGIsSetHeight_flg/1
  [DT_CAN4_SG_PTG1] -> bus_selector6/1
  bus_selector6/1 -> PTGOpenRatio/1(PTG_Open_Ratio)  "<CAN4_PTG_Open_Ratio>"
  PTGOpenRatio/1(VHAL_PTGOpenRatio_pct) -> VHAL_PTGOpenRatio_pct/1
  [DT_CAN4_SG_PTG1] -> bus_selector7/1
  bus_selector7/1 -> PTGRDILSta/1(PTG_RDIL_Sta)  "<CAN4_PTG_RDIL_Sta>"
  PTGRDILSta/1(VHAL_PTGRDILSta_enum) -> VHAL_PTGRDILSta_enum/1
  [DT_CAN4_SG_PTG1] -> bus_selector8/1
  bus_selector8/1 -> PTGSWVer/1(PTG_SW_Ver)  "<CAN4_PTG_SW_Ver>"
  PTGSWVer/1(VHAL_PTGSWVer_enum) -> VHAL_PTGSWVer_enum/1
  [DT_CAN4_SG_PTG1] -> bus_selector9/1
  bus_selector9/1 -> PTGSysSta/1(PTG_Sys_Sta)  "<CAN4_PTG_Sys_Sta>"
  PTGSysSta/1(VHAL_PTGSysSta_enum) -> VHAL_PTGSysSta_enum/1

== system halin/HAL_IN/CAN4/VHAL_CANMsgInvalidBodyZoneDR1_flg ==
  Cast To Boolean13 : DataTypeConversion  OutDataTypeStr=boolean
  Constant : Constant  Value=TRUE
  Latch13 : hcu_lib/Basic_Blocks/Latch
  Switch13 : Switch  Criteria=u2 ~= 0
  Unit Delay : UnitDelay  SampleTime=-1  HasFrameUpgradeWarning=on
  UnitConverter : DataTypeConversion  OutDataTypeStr=boolean
  Out : Outport
  wires:
  Constant/1 -> Switch13/3
  Unit Delay/1 -> Cast To Boolean13/1
  Cast To Boolean13/1 -> Switch13/1, Latch13/1
  Switch13/1 -> UnitConverter/1
  Latch13/1 -> Switch13/2
  UnitConverter/1 -> Unit Delay/1, Out/1  "VHAL_CANMsgInvalidBodyZoneDR1_flg"

== system halin/HAL_IN/CAN4/VHAL_CANMsgInvalidBodyZoneDR2_flg ==
  Cast To Boolean13 : DataTypeConversion  OutDataTypeStr=boolean
  Constant : Constant  Value=TRUE
  Latch13 : hcu_lib/Basic_Blocks/Latch
  Switch13 : Switch  Criteria=u2 ~= 0
  Unit Delay : UnitDelay  SampleTime=-1  HasFrameUpgradeWarning=on
  UnitConverter : DataTypeConversion  OutDataTypeStr=boolean
  Out : Outport
  wires:
  Constant/1 -> Switch13/3
  Unit Delay/1 -> Cast To Boolean13/1
  Cast To Boolean13/1 -> Switch13/1, Latch13/1
  Switch13/1 -> UnitConverter/1
  Latch13/1 -> Switch13/2
  UnitConverter/1 -> Unit Delay/1, Out/1  "VHAL_CANMsgInvalidBodyZoneDR2_flg"

== system halin/HAL_IN/CAN4/VHAL_CANMsgInvalidBodyZonePS1_flg ==
  Cast To Boolean13 : DataTypeConversion  OutDataTypeStr=boolean
  Constant : Constant  Value=TRUE
  Latch13 : hcu_lib/Basic_Blocks/Latch
  Switch13 : Switch  Criteria=u2 ~= 0
  Unit Delay : UnitDelay  SampleTime=-1  HasFrameUpgradeWarning=on
  UnitConverter : DataTypeConversion  OutDataTypeStr=boolean
  Out : Outport
  wires:
  Constant/1 -> Switch13/3
  Unit Delay/1 -> Cast To Boolean13/1
  Cast To Boolean13/1 -> Switch13/1, Latch13/1
  Switch13/1 -> UnitConverter/1
  Latch13/1 -> Switch13/2
  UnitConverter/1 -> Unit Delay/1, Out/1  "VHAL_CANMsgInvalidBodyZonePS1_flg"

== system halin/HAL_IN/CAN4/VHAL_CANMsgInvalidBodyZonePS2_flg ==
  Cast To Boolean13 : DataTypeConversion  OutDataTypeStr=boolean
  Constant : Constant  Value=TRUE
  Latch13 : hcu_lib/Basic_Blocks/Latch
  Switch13 : Switch  Criteria=u2 ~= 0
  Unit Delay : UnitDelay  SampleTime=-1  HasFrameUpgradeWarning=on
  UnitConverter : DataTypeConversion  OutDataTypeStr=boolean
  Out : Outport
  wires:
  Constant/1 -> Switch13/3
  Unit Delay/1 -> Cast To Boolean13/1
  Cast To Boolean13/1 -> Switch13/1, Latch13/1
  Switch13/1 -> UnitConverter/1
  Latch13/1 -> Switch13/2
  UnitConverter/1 -> Unit Delay/1, Out/1  "VHAL_CANMsgInvalidBodyZonePS2_flg"

== system halin/HAL_IN/CAN4/VHAL_CANMsgInvalidDKC1_flg ==
  Cast To Boolean13 : DataTypeConversion  OutDataTypeStr=boolean
  Constant : Constant  Value=TRUE
  Latch13 : hcu_lib/Basic_Blocks/Latch
  Switch13 : Switch  Criteria=u2 ~= 0
  Unit Delay : UnitDelay  SampleTime=-1  HasFrameUpgradeWarning=on
  UnitConverter : DataTypeConversion  OutDataTypeStr=boolean
  Out : Outport
  wires:
  Constant/1 -> Switch13/3
  Unit Delay/1 -> Cast To Boolean13/1
  Cast To Boolean13/1 -> Switch13/1, Latch13/1
  Switch13/1 -> UnitConverter/1
  Latch13/1 -> Switch13/2
  UnitConverter/1 -> Unit Delay/1, Out/1  "VHAL_CANMsgInvalidDKC1_flg"

== system halin/HAL_IN/CAN4/VHAL_CANMsgInvalidDKC2_flg ==
  Cast To Boolean13 : DataTypeConversion  OutDataTypeStr=boolean
  Constant : Constant  Value=TRUE
  Latch13 : hcu_lib/Basic_Blocks/Latch
  Switch13 : Switch  Criteria=u2 ~= 0
  Unit Delay : UnitDelay  SampleTime=-1  HasFrameUpgradeWarning=on
  UnitConverter : DataTypeConversion  OutDataTypeStr=boolean
  Out : Outport
  wires:
  Constant/1 -> Switch13/3
  Unit Delay/1 -> Cast To Boolean13/1
  Cast To Boolean13/1 -> Switch13/1, Latch13/1
  Switch13/1 -> UnitConverter/1
  Latch13/1 -> Switch13/2
  UnitConverter/1 -> Unit Delay/1, Out/1  "VHAL_CANMsgInvalidDKC2_flg"

== system halin/HAL_IN/CAN4/VHAL_CANMsgInvalidPTG1_flg ==
  Cast To Boolean13 : DataTypeConversion  OutDataTypeStr=boolean
  Constant : Constant  Value=TRUE
  Latch13 : hcu_lib/Basic_Blocks/Latch
  Switch13 : Switch  Criteria=u2 ~= 0
  Unit Delay : UnitDelay  SampleTime=-1  HasFrameUpgradeWarning=on
  UnitConverter : DataTypeConversion  OutDataTypeStr=boolean
  Out : Outport
  wires:
  Constant/1 -> Switch13/3
  Unit Delay/1 -> Cast To Boolean13/1
  Cast To Boolean13/1 -> Switch13/1, Latch13/1
  Switch13/1 -> UnitConverter/1
  Latch13/1 -> Switch13/2
  UnitConverter/1 -> Unit Delay/1, Out/1  "VHAL_CANMsgInvalidPTG1_flg"

== system halin/HAL_IN/CAN4/VHAL_CANMsgInvalidZONEDR1_flg ==
  Cast To Boolean13 : DataTypeConversion  OutDataTypeStr=boolean
  Constant : Constant  Value=TRUE
  Latch13 : hcu_lib/Basic_Blocks/Latch
  Switch13 : Switch  Criteria=u2 ~= 0
  Unit Delay : UnitDelay  SampleTime=-1  HasFrameUpgradeWarning=on
  UnitConverter : DataTypeConversion  OutDataTypeStr=boolean
  Out : Outport
  wires:
  Constant/1 -> Switch13/3
  Unit Delay/1 -> Cast To Boolean13/1
  Cast To Boolean13/1 -> Switch13/1, Latch13/1
  Switch13/1 -> UnitConverter/1
  Latch13/1 -> Switch13/2
  UnitConverter/1 -> Unit Delay/1, Out/1  "VHAL_CANMsgInvalidZONEDR1_flg"

== system halin/HAL_IN/CAN4/VHAL_CANMsgInvalidZONEDRVCU_flg ==
  Cast To Boolean13 : DataTypeConversion  OutDataTypeStr=boolean
  Constant : Constant  Value=TRUE
  Latch13 : hcu_lib/Basic_Blocks/Latch
  Switch13 : Switch  Criteria=u2 ~= 0
  Unit Delay : UnitDelay  SampleTime=-1  HasFrameUpgradeWarning=on
  UnitConverter : DataTypeConversion  OutDataTypeStr=boolean
  Out : Outport
  wires:
  Constant/1 -> Switch13/3
  Unit Delay/1 -> Cast To Boolean13/1
  Cast To Boolean13/1 -> Switch13/1, Latch13/1
  Switch13/1 -> UnitConverter/1
  Latch13/1 -> Switch13/2
  UnitConverter/1 -> Unit Delay/1, Out/1  "VHAL_CANMsgInvalidZONEDRVCU_flg"

== system halin/HAL_IN/CAN4/VHAL_CANMsgInvalidZONEFR1_flg ==
  Cast To Boolean13 : DataTypeConversion  OutDataTypeStr=boolean
  Constant : Constant  Value=TRUE
  Latch13 : hcu_lib/Basic_Blocks/Latch
  Switch13 : Switch  Criteria=u2 ~= 0
  Unit Delay : UnitDelay  SampleTime=-1  HasFrameUpgradeWarning=on
  UnitConverter : DataTypeConversion  OutDataTypeStr=boolean
  Out : Outport
  wires:
  Constant/1 -> Switch13/3
  Unit Delay/1 -> Cast To Boolean13/1
  Cast To Boolean13/1 -> Switch13/1, Latch13/1
  Switch13/1 -> UnitConverter/1
  Latch13/1 -> Switch13/2
  UnitConverter/1 -> Unit Delay/1, Out/1  "VHAL_CANMsgInvalidZONEFR1_flg"

== system halin/HAL_IN/CAN4/VHAL_CANMsgInvalidZONEFRVCU_flg ==
  Cast To Boolean13 : DataTypeConversion  OutDataTypeStr=boolean
  Constant : Constant  Value=TRUE
  Latch13 : hcu_lib/Basic_Blocks/Latch
  Switch13 : Switch  Criteria=u2 ~= 0
  Unit Delay : UnitDelay  SampleTime=-1  HasFrameUpgradeWarning=on
  UnitConverter : DataTypeConversion  OutDataTypeStr=boolean
  Out : Outport
  wires:
  Constant/1 -> Switch13/3
  Unit Delay/1 -> Cast To Boolean13/1
  Cast To Boolean13/1 -> Switch13/1, Latch13/1
  Switch13/1 -> UnitConverter/1
  Latch13/1 -> Switch13/2
  UnitConverter/1 -> Unit Delay/1, Out/1  "VHAL_CANMsgInvalidZONEFRVCU_flg"

== system halin/HAL_IN/CAN4/VHAL_CANMsgInvalidzGWAPTC1_flg ==
  Cast To Boolean13 : DataTypeConversion  OutDataTypeStr=boolean
  Constant : Constant  Value=TRUE
  Latch13 : hcu_lib/Basic_Blocks/Latch
  Switch13 : Switch  Criteria=u2 ~= 0
  Unit Delay : UnitDelay  SampleTime=-1  HasFrameUpgradeWarning=on
  UnitConverter : DataTypeConversion  OutDataTypeStr=boolean
  Out : Outport
  wires:
  Constant/1 -> Switch13/3
  Unit Delay/1 -> Cast To Boolean13/1
  Cast To Boolean13/1 -> Switch13/1, Latch13/1
  Switch13/1 -> UnitConverter/1
  Latch13/1 -> Switch13/2
  UnitConverter/1 -> Unit Delay/1, Out/1  "VHAL_CANMsgInvalidzGWAPTC1_flg"

== system halin/HAL_IN/CAN4/VHAL_CANMsgInvalidzGWCANFr1_flg ==
  Cast To Boolean13 : DataTypeConversion  OutDataTypeStr=boolean
  Constant : Constant  Value=TRUE
  Latch13 : hcu_lib/Basic_Blocks/Latch
  Switch13 : Switch  Criteria=u2 ~= 0
  Unit Delay : UnitDelay  SampleTime=-1  HasFrameUpgradeWarning=on
  UnitConverter : DataTypeConversion  OutDataTypeStr=boolean
  Out : Outport
  wires:
  Constant/1 -> Switch13/3
  Unit Delay/1 -> Cast To Boolean13/1
  Cast To Boolean13/1 -> Switch13/1, Latch13/1
  Switch13/1 -> UnitConverter/1
  Latch13/1 -> Switch13/2
  UnitConverter/1 -> Unit Delay/1, Out/1  "VHAL_CANMsgInvalidzGWCANFr1_flg"

== system halin/HAL_IN/CAN4/VHAL_CANMsgInvalidzGWLINDr1_flg ==
  Cast To Boolean13 : DataTypeConversion  OutDataTypeStr=boolean
  Constant : Constant  Value=TRUE
  Latch13 : hcu_lib/Basic_Blocks/Latch
  Switch13 : Switch  Criteria=u2 ~= 0
  Unit Delay : UnitDelay  SampleTime=-1  HasFrameUpgradeWarning=on
  UnitConverter : DataTypeConversion  OutDataTypeStr=boolean
  Out : Outport
  wires:
  Constant/1 -> Switch13/3
  Unit Delay/1 -> Cast To Boolean13/1
  Cast To Boolean13/1 -> Switch13/1, Latch13/1
  Switch13/1 -> UnitConverter/1
  Latch13/1 -> Switch13/2
  UnitConverter/1 -> Unit Delay/1, Out/1  "VHAL_CANMsgInvalidzGWLINDr1_flg"

== system halin/HAL_IN/CAN4/VHAL_CANMsgInvalidzGWLINDr2_flg ==
  Cast To Boolean13 : DataTypeConversion  OutDataTypeStr=boolean
  Constant : Constant  Value=TRUE
  Latch13 : hcu_lib/Basic_Blocks/Latch
  Switch13 : Switch  Criteria=u2 ~= 0
  Unit Delay : UnitDelay  SampleTime=-1  HasFrameUpgradeWarning=on
  UnitConverter : DataTypeConversion  OutDataTypeStr=boolean
  Out : Outport
  wires:
  Constant/1 -> Switch13/3
  Unit Delay/1 -> Cast To Boolean13/1
  Cast To Boolean13/1 -> Switch13/1, Latch13/1
  Switch13/1 -> UnitConverter/1
  Latch13/1 -> Switch13/2
  UnitConverter/1 -> Unit Delay/1, Out/1  "VHAL_CANMsgInvalidzGWLINDr2_flg"

== system halin/HAL_IN/CAN4/VHAL_CANMsgInvalidzGWLINFr1_flg ==
  Cast To Boolean13 : DataTypeConversion  OutDataTypeStr=boolean
  Constant : Constant  Value=TRUE
  Latch13 : hcu_lib/Basic_Blocks/Latch
  Switch13 : Switch  Criteria=u2 ~= 0
  Unit Delay : UnitDelay  SampleTime=-1  HasFrameUpgradeWarning=on
  UnitConverter : DataTypeConversion  OutDataTypeStr=boolean
  Out : Outport
  wires:
  Constant/1 -> Switch13/3
  Unit Delay/1 -> Cast To Boolean13/1
  Cast To Boolean13/1 -> Switch13/1, Latch13/1
  Switch13/1 -> UnitConverter/1
  Latch13/1 -> Switch13/2
  UnitConverter/1 -> Unit Delay/1, Out/1  "VHAL_CANMsgInvalidzGWLINFr1_flg"

== system halin/HAL_IN/CAN4/VHAL_CANMsgInvalidzGWLINFr2_flg ==
  Cast To Boolean13 : DataTypeConversion  OutDataTypeStr=boolean
  Constant : Constant  Value=TRUE
  Latch13 : hcu_lib/Basic_Blocks/Latch
  Switch13 : Switch  Criteria=u2 ~= 0
  Unit Delay : UnitDelay  SampleTime=-1  HasFrameUpgradeWarning=on
  UnitConverter : DataTypeConversion  OutDataTypeStr=boolean
  Out : Outport
  wires:
  Constant/1 -> Switch13/3
  Unit Delay/1 -> Cast To Boolean13/1
  Cast To Boolean13/1 -> Switch13/1, Latch13/1
  Switch13/1 -> UnitConverter/1
  Latch13/1 -> Switch13/2
  UnitConverter/1 -> Unit Delay/1, Out/1  "VHAL_CANMsgInvalidzGWLINFr2_flg"

== system halin/HAL_IN/CAN4/VHAL_CANMsgInvalidzGWSEAT1_flg ==
  Cast To Boolean13 : DataTypeConversion  OutDataTypeStr=boolean
  Constant : Constant  Value=TRUE
  Latch13 : hcu_lib/Basic_Blocks/Latch
  Switch13 : Switch  Criteria=u2 ~= 0
  Unit Delay : UnitDelay  SampleTime=-1  HasFrameUpgradeWarning=on
  UnitConverter : DataTypeConversion  OutDataTypeStr=boolean
  Out : Outport
  wires:
  Constant/1 -> Switch13/3
  Unit Delay/1 -> Cast To Boolean13/1
  Cast To Boolean13/1 -> Switch13/1, Latch13/1
  Switch13/1 -> UnitConverter/1
  Latch13/1 -> Switch13/2
  UnitConverter/1 -> Unit Delay/1, Out/1  "VHAL_CANMsgInvalidzGWSEAT1_flg"

== system halin/HAL_IN/CAN4/ZONE_DR1 ==
  DT_CAN4_SG_ZONE_DR1 : Inport
  DrLockSta : Subsystem
  MIRRORFOLDSW : Subsystem
  RLTurnLPErr : Subsystem
  RLTurnLampC : Subsystem
  RRTurnLPErr : Subsystem
  RRTurnLampC : Subsystem
  RWiperAS : Subsystem
  RWiperProtection : Subsystem
  bus_selector : BusSelector  OutputSignals=CAN4_DrLockSta
  bus_selector1 : BusSelector  OutputSignals=CAN4_MIRROR_FOLD_SW
  bus_selector2 : BusSelector  OutputSignals=CAN4_RLTurnLPErr
  bus_selector3 : BusSelector  OutputSignals=CAN4_RLTurnLampC
  bus_selector4 : BusSelector  OutputSignals=CAN4_RRTurnLPErr
  bus_selector5 : BusSelector  OutputSignals=CAN4_RRTurnLampC
  bus_selector6 : BusSelector  OutputSignals=CAN4_RWiperAS
  bus_selector7 : BusSelector  OutputSignals=CAN4_RWiperProtection
  VHAL_DrLockSta_flg : Outport
  VHAL_MIRRORFOLDSW_flg : Outport  Port=2
  VHAL_RLTurnLPErr_flg : Outport  Port=3
  VHAL_RLTurnLampC_mA : Outport  Port=4
  VHAL_RRTurnLPErr_flg : Outport  Port=5
  VHAL_RRTurnLampC_mA : Outport  Port=6
  VHAL_RWiperAS_flg : Outport  Port=7
  VHAL_RWiperProtection_flg : Outport  Port=8
  wires:
  DT_CAN4_SG_ZONE_DR1/1 -> [DT_CAN4_SG_ZONE_DR1]
  [DT_CAN4_SG_ZONE_DR1] -> bus_selector/1
  bus_selector/1 -> DrLockSta/1(DrLockSta)  "<CAN4_DrLockSta>"
  DrLockSta/1(VHAL_DrLockSta_flg) -> VHAL_DrLockSta_flg/1
  [DT_CAN4_SG_ZONE_DR1] -> bus_selector1/1
  bus_selector1/1 -> MIRRORFOLDSW/1(MIRROR_FOLD_SW)  "<CAN4_MIRROR_FOLD_SW>"
  MIRRORFOLDSW/1(VHAL_MIRRORFOLDSW_flg) -> VHAL_MIRRORFOLDSW_flg/1
  [DT_CAN4_SG_ZONE_DR1] -> bus_selector2/1
  bus_selector2/1 -> RLTurnLPErr/1(RLTurnLPErr)  "<CAN4_RLTurnLPErr>"
  RLTurnLPErr/1(VHAL_RLTurnLPErr_flg) -> VHAL_RLTurnLPErr_flg/1
  [DT_CAN4_SG_ZONE_DR1] -> bus_selector3/1
  bus_selector3/1 -> RLTurnLampC/1(RLTurnLampC)  "<CAN4_RLTurnLampC>"
  RLTurnLampC/1(VHAL_RLTurnLampC_mA) -> VHAL_RLTurnLampC_mA/1
  [DT_CAN4_SG_ZONE_DR1] -> bus_selector4/1
  bus_selector4/1 -> RRTurnLPErr/1(RRTurnLPErr)  "<CAN4_RRTurnLPErr>"
  RRTurnLPErr/1(VHAL_RRTurnLPErr_flg) -> VHAL_RRTurnLPErr_flg/1
  [DT_CAN4_SG_ZONE_DR1] -> bus_selector5/1
  bus_selector5/1 -> RRTurnLampC/1(RRTurnLampC)  "<CAN4_RRTurnLampC>"
  RRTurnLampC/1(VHAL_RRTurnLampC_mA) -> VHAL_RRTurnLampC_mA/1
  [DT_CAN4_SG_ZONE_DR1] -> bus_selector6/1
  bus_selector6/1 -> RWiperAS/1(RWiperAS)  "<CAN4_RWiperAS>"
  RWiperAS/1(VHAL_RWiperAS_flg) -> VHAL_RWiperAS_flg/1
  [DT_CAN4_SG_ZONE_DR1] -> bus_selector7/1
  bus_selector7/1 -> RWiperProtection/1(RWiperProtection)  "<CAN4_RWiperProtection>"
  RWiperProtection/1(VHAL_RWiperProtection_flg) -> VHAL_RWiperProtection_flg/1

== system halin/HAL_IN/CAN4/ZONE_DR_VCU ==
  DT_CAN4_SG_ZONE_DR_VCU : Inport
  BlowerErr : Subsystem
  DrPMMLVOutPErrLmp : Subsystem
  DrPMMSysErrLmp : Subsystem
  DrSCPSysErrLmp : Subsystem
  DrStdAErrSta : Subsystem
  LeftHallPos : Subsystem
  SolarL : Subsystem
  SolarLErr : Subsystem
  SolarR : Subsystem
  SolarRErr : Subsystem
  TFaceL : Subsystem
  TFaceLErr : Subsystem
  TFaceR : Subsystem
  TFaceRErr : Subsystem
  TFaceRr : Subsystem
  TFaceRrErr : Subsystem
  TFootL : Subsystem
  TFootLErr : Subsystem
  TFootR : Subsystem
  TFootRErr : Subsystem
  TFootRr : Subsystem
  TFootRrErr : Subsystem
  Tevap : Subsystem
  TevapErr : Subsystem
  Tincar : Subsystem
  TincarErr : Subsystem
  ZoneDrMalfunLevel : Subsystem
  bus_selector : BusSelector  OutputSignals=CAN4_Blower_Err
  bus_selector1 : BusSelector  OutputSignals=CAN4_DrPMMLVOutPErrLmp
  bus_selector10 : BusSelector  OutputSignals=CAN4_T_Face_L
  bus_selector11 : BusSelector  OutputSignals=CAN4_T_Face_L_Err
  bus_selector12 : BusSelector  OutputSignals=CAN4_T_Face_R
  bus_selector13 : BusSelector  OutputSignals=CAN4_T_Face_R_Err
  bus_selector14 : BusSelector  OutputSignals=CAN4_T_Face_Rr
  bus_selector15 : BusSelector  OutputSignals=CAN4_T_Face_Rr_Err
  bus_selector16 : BusSelector  OutputSignals=CAN4_T_Foot_L
  bus_selector17 : BusSelector  OutputSignals=CAN4_T_Foot_L_Err
  bus_selector18 : BusSelector  OutputSignals=CAN4_T_Foot_R
  bus_selector19 : BusSelector  OutputSignals=CAN4_T_Foot_R_Err
  bus_selector2 : BusSelector  OutputSignals=CAN4_DrPMMSysErrLmp
  bus_selector20 : BusSelector  OutputSignals=CAN4_T_Foot_Rr
  bus_selector21 : BusSelector  OutputSignals=CAN4_T_Foot_Rr_Err
  bus_selector22 : BusSelector  OutputSignals=CAN4_Tevap
  bus_selector23 : BusSelector  OutputSignals=CAN4_Tevap_Err
  bus_selector24 : BusSelector  OutputSignals=CAN4_Tincar
  bus_selector25 : BusSelector  OutputSignals=CAN4_Tincar_Err
  bus_selector26 : BusSelector  OutputSignals=CAN4_ZoneDrMalfunLevel
  bus_selector3 : BusSelector  OutputSignals=CAN4_DrSCPSysErrLmp
  bus_selector4 : BusSelector  OutputSignals=CAN4_DrStdAErrSta
  bus_selector5 : BusSelector  OutputSignals=CAN4_LeftHall_Pos
  bus_selector6 : BusSelector  OutputSignals=CAN4_SolarL
  bus_selector7 : BusSelector  OutputSignals=CAN4_SolarL_Err
  bus_selector8 : BusSelector  OutputSignals=CAN4_SolarR
  bus_selector9 : BusSelector  OutputSignals=CAN4_SolarR_Err
  VHAL_BlowerErr_enum : Outport
  VHAL_DrPMMLVOutPErrLmp_flg : Outport  Port=2
  VHAL_DrPMMSysErrLmp_flg : Outport  Port=3
  VHAL_DrSCPSysErrLmp_flg : Outport  Port=4
  VHAL_DrStdAErrSta_flg : Outport  Port=5
  VHAL_LeftHallPos_enum : Outport  Port=6
  VHAL_SolarL_W : Outport  Port=7
  VHAL_SolarLErr_enum : Outport  Port=8
  VHAL_SolarR_W : Outport  Port=9
  VHAL_SolarRErr_enum : Outport  Port=10
  VHAL_TFaceL_C : Outport  Port=11
  VHAL_TFaceLErr_enum : Outport  Port=12
  VHAL_TFaceR_C : Outport  Port=13
  VHAL_TFaceRErr_enum : Outport  Port=14
  VHAL_TFaceRr_C : Outport  Port=15
  VHAL_TFaceRrErr_enum : Outport  Port=16
  VHAL_TFootL_C : Outport  Port=17
  VHAL_TFootLErr_enum : Outport  Port=18
  VHAL_TFootR_C : Outport  Port=19
  VHAL_TFootRErr_enum : Outport  Port=20
  VHAL_TFootRr_C : Outport  Port=21
  VHAL_TFootRrErr_enum : Outport  Port=22
  VHAL_Tevap_C : Outport  Port=23
  VHAL_TevapErr_enum : Outport  Port=24
  VHAL_Tincar_C : Outport  Port=25
  VHAL_TincarErr_enum : Outport  Port=26
  VHAL_ZoneDrMalfunLevel_enum : Outport  Port=27
  wires:
  DT_CAN4_SG_ZONE_DR_VCU/1 -> [DT_CAN4_SG_ZONE_DR_VCU]
  [DT_CAN4_SG_ZONE_DR_VCU] -> bus_selector/1
  bus_selector/1 -> BlowerErr/1(Blower_Err)  "<CAN4_Blower_Err>"
  BlowerErr/1(VHAL_BlowerErr_enum) -> VHAL_BlowerErr_enum/1
  [DT_CAN4_SG_ZONE_DR_VCU] -> bus_selector1/1
  bus_selector1/1 -> DrPMMLVOutPErrLmp/1(DrPMMLVOutPErrLmp)  "<CAN4_DrPMMLVOutPErrLmp>"
  DrPMMLVOutPErrLmp/1(VHAL_DrPMMLVOutPErrLmp_flg) -> VHAL_DrPMMLVOutPErrLmp_flg/1
  [DT_CAN4_SG_ZONE_DR_VCU] -> bus_selector2/1
  bus_selector2/1 -> DrPMMSysErrLmp/1(DrPMMSysErrLmp)  "<CAN4_DrPMMSysErrLmp>"
  DrPMMSysErrLmp/1(VHAL_DrPMMSysErrLmp_flg) -> VHAL_DrPMMSysErrLmp_flg/1
  [DT_CAN4_SG_ZONE_DR_VCU] -> bus_selector3/1
  bus_selector3/1 -> DrSCPSysErrLmp/1(DrSCPSysErrLmp)  "<CAN4_DrSCPSysErrLmp>"
  DrSCPSysErrLmp/1(VHAL_DrSCPSysErrLmp_flg) -> VHAL_DrSCPSysErrLmp_flg/1
  [DT_CAN4_SG_ZONE_DR_VCU] -> bus_selector4/1
  bus_selector4/1 -> DrStdAErrSta/1(DrStdAErrSta)  "<CAN4_DrStdAErrSta>"
  DrStdAErrSta/1(VHAL_DrStdAErrSta_flg) -> VHAL_DrStdAErrSta_flg/1
  [DT_CAN4_SG_ZONE_DR_VCU] -> bus_selector5/1
  bus_selector5/1 -> LeftHallPos/1(LeftHall_Pos)  "<CAN4_LeftHall_Pos>"
  LeftHallPos/1(VHAL_LeftHallPos_enum) -> VHAL_LeftHallPos_enum/1
  [DT_CAN4_SG_ZONE_DR_VCU] -> bus_selector6/1
  bus_selector6/1 -> SolarL/1(SolarL)  "<CAN4_SolarL>"
  SolarL/1(VHAL_SolarL_W) -> VHAL_SolarL_W/1
  [DT_CAN4_SG_ZONE_DR_VCU] -> bus_selector7/1
  bus_selector7/1 -> SolarLErr/1(SolarL_Err)  "<CAN4_SolarL_Err>"
  SolarLErr/1(VHAL_SolarLErr_enum) -> VHAL_SolarLErr_enum/1
  [DT_CAN4_SG_ZONE_DR_VCU] -> bus_selector8/1
  bus_selector8/1 -> SolarR/1(SolarR)  "<CAN4_SolarR>"
  SolarR/1(VHAL_SolarR_W) -> VHAL_SolarR_W/1
  [DT_CAN4_SG_ZONE_DR_VCU] -> bus_selector9/1
  bus_selector9/1 -> SolarRErr/1(SolarR_Err)  "<CAN4_SolarR_Err>"
  SolarRErr/1(VHAL_SolarRErr_enum) -> VHAL_SolarRErr_enum/1
  [DT_CAN4_SG_ZONE_DR_VCU] -> bus_selector10/1
  bus_selector10/1 -> TFaceL/1(T_Face_L)  "<CAN4_T_Face_L>"
  TFaceL/1(VHAL_TFaceL_C) -> VHAL_TFaceL_C/1
  [DT_CAN4_SG_ZONE_DR_VCU] -> bus_selector11/1
  bus_selector11/1 -> TFaceLErr/1(T_Face_L_Err)  "<CAN4_T_Face_L_Err>"
  TFaceLErr/1(VHAL_TFaceLErr_enum) -> VHAL_TFaceLErr_enum/1
  [DT_CAN4_SG_ZONE_DR_VCU] -> bus_selector12/1
  bus_selector12/1 -> TFaceR/1(T_Face_R)  "<CAN4_T_Face_R>"
  TFaceR/1(VHAL_TFaceR_C) -> VHAL_TFaceR_C/1
  [DT_CAN4_SG_ZONE_DR_VCU] -> bus_selector13/1
  bus_selector13/1 -> TFaceRErr/1(T_Face_R_Err)  "<CAN4_T_Face_R_Err>"
  TFaceRErr/1(VHAL_TFaceRErr_enum) -> VHAL_TFaceRErr_enum/1
  [DT_CAN4_SG_ZONE_DR_VCU] -> bus_selector14/1
  bus_selector14/1 -> TFaceRr/1(T_Face_Rr)  "<CAN4_T_Face_Rr>"
  TFaceRr/1(VHAL_TFaceRr_C) -> VHAL_TFaceRr_C/1
  [DT_CAN4_SG_ZONE_DR_VCU] -> bus_selector15/1
  bus_selector15/1 -> TFaceRrErr/1(T_Face_Rr_Err)  "<CAN4_T_Face_Rr_Err>"
  TFaceRrErr/1(VHAL_TFaceRrErr_enum) -> VHAL_TFaceRrErr_enum/1
  [DT_CAN4_SG_ZONE_DR_VCU] -> bus_selector16/1
  bus_selector16/1 -> TFootL/1(T_Foot_L)  "<CAN4_T_Foot_L>"
  TFootL/1(VHAL_TFootL_C) -> VHAL_TFootL_C/1
  [DT_CAN4_SG_ZONE_DR_VCU] -> bus_selector17/1
  bus_selector17/1 -> TFootLErr/1(T_Foot_L_Err)  "<CAN4_T_Foot_L_Err>"
  TFootLErr/1(VHAL_TFootLErr_enum) -> VHAL_TFootLErr_enum/1
  [DT_CAN4_SG_ZONE_DR_VCU] -> bus_selector18/1
  bus_selector18/1 -> TFootR/1(T_Foot_R)  "<CAN4_T_Foot_R>"
  TFootR/1(VHAL_TFootR_C) -> VHAL_TFootR_C/1
  [DT_CAN4_SG_ZONE_DR_VCU] -> bus_selector19/1
  bus_selector19/1 -> TFootRErr/1(T_Foot_R_Err)  "<CAN4_T_Foot_R_Err>"
  TFootRErr/1(VHAL_TFootRErr_enum) -> VHAL_TFootRErr_enum/1
  [DT_CAN4_SG_ZONE_DR_VCU] -> bus_selector20/1
  bus_selector20/1 -> TFootRr/1(T_Foot_Rr)  "<CAN4_T_Foot_Rr>"
  TFootRr/1(VHAL_TFootRr_C) -> VHAL_TFootRr_C/1
  [DT_CAN4_SG_ZONE_DR_VCU] -> bus_selector21/1
  bus_selector21/1 -> TFootRrErr/1(T_Foot_Rr_Err)  "<CAN4_T_Foot_Rr_Err>"
  TFootRrErr/1(VHAL_TFootRrErr_enum) -> VHAL_TFootRrErr_enum/1
  [DT_CAN4_SG_ZONE_DR_VCU] -> bus_selector22/1
  bus_selector22/1 -> Tevap/1(Tevap)  "<CAN4_Tevap>"
  Tevap/1(VHAL_Tevap_C) -> VHAL_Tevap_C/1
  [DT_CAN4_SG_ZONE_DR_VCU] -> bus_selector23/1
  bus_selector23/1 -> TevapErr/1(Tevap_Err)  "<CAN4_Tevap_Err>"
  TevapErr/1(VHAL_TevapErr_enum) -> VHAL_TevapErr_enum/1
  [DT_CAN4_SG_ZONE_DR_VCU] -> bus_selector24/1
  bus_selector24/1 -> Tincar/1(Tincar)  "<CAN4_Tincar>"
  Tincar/1(VHAL_Tincar_C) -> VHAL_Tincar_C/1
  [DT_CAN4_SG_ZONE_DR_VCU] -> bus_selector25/1
  bus_selector25/1 -> TincarErr/1(Tincar_Err)  "<CAN4_Tincar_Err>"
  TincarErr/1(VHAL_TincarErr_enum) -> VHAL_TincarErr_enum/1
  [DT_CAN4_SG_ZONE_DR_VCU] -> bus_selector26/1
  bus_selector26/1 -> ZoneDrMalfunLevel/1(ZoneDrMalfunLevel)  "<CAN4_ZoneDrMalfunLevel>"
  ZoneDrMalfunLevel/1(VHAL_ZoneDrMalfunLevel_enum) -> VHAL_ZoneDrMalfunLevel_enum/1
